simulink model "Lab2_Simulink_Design_Part3_1"  (R2020a)
settings: Solver=VariableStepAuto  StartTime=0.0  StopTime=10.0  RelTol=1e-3
settings Model: Creator=mati1  LastModifiedBy=mati1

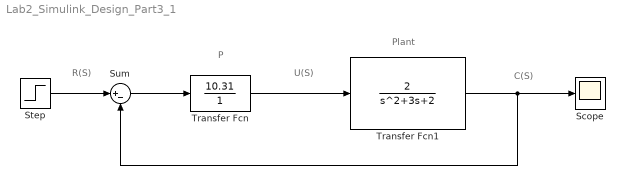
== system Lab2_Simulink_Design_Part3_1 ==
  note: R(S)
  note: P
  note: C(S)
  note: U(S)
  note: Plant
  Scope : Scope
  Step : Step  Before=1  SampleTime=0
  Sum : Sum  Inputs=|+-
  Transfer Fcn : TransferFcn  Numerator=[10.31]  Denominator=[1]
  Transfer Fcn1 : TransferFcn  Numerator=[2]  Denominator=[1 3 2]
  wires:
  Sum/1 -> Transfer Fcn/1
  Transfer Fcn/1 -> Transfer Fcn1/1
  Step/1 -> Sum/1
  Transfer Fcn1/1 -> Scope/1, Sum/2
